simulink model "uplink_8c4r"  (Simulink 8.7)
settings: Solver=VariableStepDiscrete  StartTime=0.0  StopTime=20000  RelTol=1e-3
PreLoadFcn:
  | % Run the setup script when the model is opened
  | setup_uplink_8c4r;
InitFcn:
  | % Run the setup script again just before the
  | % model is run, so that any updates made
  | % after opening are applied.
  | setup_uplink_8c4r;
  | %% DSPBuilder Start
  | alt_dspbuilder_update_model(bdroot)
  | %% DSPBuilder End
undefined symbols (not defined in the file or in its folder): DDC_Lineup_param
libraries: pipereg_lib x8, DSPBABase x7, ddc_mixer_lib x4, hddc_lib x4, lddc_lib x4, simulink x1
Description:
  | DSP Builder Advanced Template for Template Design implementing ModelIP designs
settings Model: Creator=mjervis  LastModifiedBy=5g
settings DataIOCC: SignalLoggingSaveFormat=ModelDataLogs
settings OptimizationCC: ExpressionDepthLimit=2147483647
settings DebuggingCC: SolverPrmCheckMsg=warning  InheritedTsInSrcMsg=none  IntegerOverflowMsg=none  ParameterOverflowMsg=none  FcnCallInpInsideContextMsg=UseLocalSettings  StateNameClashWarn=warning  IntegerSaturationMsg=none
settings GRTTargetCC: CombineOutputUpdateFcns=off  GRTInterface=on
settings ConfigComp: CovSFcnEnable=off

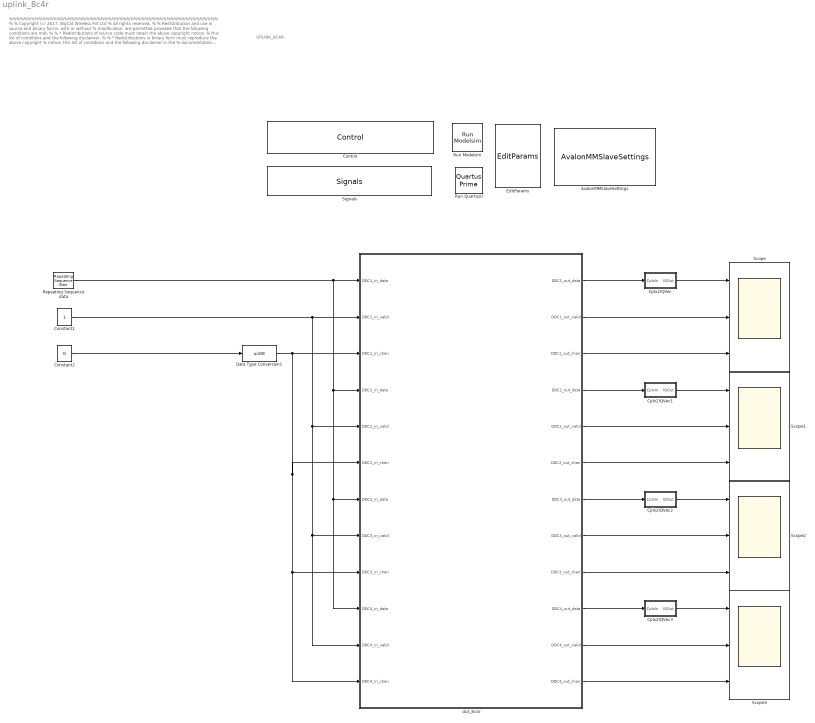
== system uplink_8c4r ==
  note: %%%%%%%%%%%%%%%%%%%%%%%%%%%%%%%%%%%%%%%%%%%%%%%%%%%%%%%%%
      |  %
      |  % Copyright (c) 2017, BigCat Wireless Pvt Ltd
      |  % All rights reserved.
      |  %
      |  % Redistribution and use in source and binary forms, with or without
      |  % modification, are permitted provided that the following conditions are met:
      |  %
      |  %     * Redistributions of source code must retain the above copyright notice,
      |  %       this list of conditions and the following disclaimer.
      |  %
      |  %     * Redistributions in binary form must reproduce the above copyright
      |  %       notice, this list of conditions and the following disclaimer in the
      |  %       documentation and/or other materials provided with the distribution.
      |  %
      |  %     * Neither the name of the copyright holder nor the names of its contributors
      |  %       may be used to endorse or promote products derived from this software
      |  %       without specific prior written permission.
      |  %
      |  %
      |  %
      |  % THIS SOFTWARE IS PROVIDED BY THE COPYRIGHT HOLDERS AND CONTRIBUTORS "AS IS"
      |  % AND ANY EXPRESS OR IMPLIED WARRANTIES, INCLUDING, BUT NOT LIMITED TO, THE
      |  % IMPLIED WARRANTIES OF MERCHANTABILITY AND FITNESS FOR A PARTICULAR PURPOSE ARE
      |  % DISCLAIMED. IN NO EVENT SHALL THE COPYRIGHT HOLDER OR CONTRIBUTORS BE LIABLE
      |  % FOR ANY DIRECT, INDIRECT, INCIDENTAL, SPECIAL, EXEMPLARY, OR CONSEQUENTIAL
      |  % DAMAGES (INCLUDING, BUT NOT LIMITED TO, PROCUREMENT OF SUBSTITUTE GOODS OR
      |  % SERVICES; LOSS OF USE, DATA, OR PROFITS; OR BUSINESS INTERRUPTION) HOWEVER
      |  % CAUSED AND ON ANY THEORY OF LIABILITY, WHETHER IN CONTRACT, STRICT LIABILITY,
      |  % OR TORT (INCLUDING NEGLIGENCE OR OTHERWISE) ARISING IN ANY WAY OUT OF THE USE
      |  % OF THIS SOFTWARE, EVEN IF ADVISED OF THE POSSIBILITY OF SUCH DAMAGE.
      |  %
      |   %%%%%%%%%%%%%%%%%%%%%%%%%%%%%%%%%%%%%%%%%%%%%%%%%%%%%%%%%%
  note: UPLINK_8C4R
  AvalonMMSlaveSettings : DSPBABase/AvalonMMSlaveSettings
  Constant1 : Constant  OutDataTypeStr=boolean
  Constant2 : Constant  Value=0  OutDataTypeStr=boolean
  Control : DSPBABase/Control  generate=on  language=VHDL  destination=./rtl  destination_gui=./rtl  make_full_path=off  path_is_relative=on  autotestbench=off  signaldepth=2  coveragetestbench=on  logs=off  spacewidth=2  spacenum=1  addrwidth=11  datawidth=32  dataendian=Big Endian  hierarchicalnames=off  ramThresholdBits=-1  distRamThresholdBits=-1  mlabThresholdBits=-1  hardMultiplierThresholdLuts=-1  version=20090407  errorOnChanMismatch=1  errorOnGPIOMismatch=0  importModelsimResults=0  cycleAccurate=off  reinterpretCastMult=off  paramFile=uplink_8c4r_params.xml
  Cplx2IQVec : Subsystem
  Cplx2IQVec1 : Subsystem
  Cplx2IQVec2 : Subsystem
  Cplx2IQVec3 : Subsystem
  Data Type Conversion1 : DataTypeConversion  OutDataTypeStr=uint8
  EditParams : DSPBABase/EditParams  version=20090407
  Repeating Sequence data : simulink/Sources/Repeating Sequence Stair  OutValues=DDC_Lineup_param.inputdata.'  tsamp=1  OutMin=[]  OutMax=[]  OutDataTypeStr=fixdt(1,16,15)  OutputDataTypeScalingMode=Specify via dialog  OutDataType=fixdt(1,16,15)  ConRadixGroup=Best Precision: Vector-wise  OutScaling=[]
  Run Modelsim : DSPBABase/Run Modelsim  version=20090407
  "Run QuartusII " : DSPBABase/Quartus Prime  version=20090407
  Scope{,1..3} (4 alike) : Scope  NumInputPorts=3
  Signals : DSPBABase/Signals  clk=clk  freq=DDC_Lineup_param.ClockRate  margin=DDC_Lineup_param.ClockMargin  rst=areset  rstactive=High  bus=bus  enbusclock=on  busfreq=61.44  bussync=on  version=20090407
  dut_8c4r : Subsystem
  wires:
  Constant2/1 -> Data Type Conversion1/1
  Repeating Sequence data/1 -> dut_8c4r/10(DDC4_in_data), dut_8c4r/7(DDC3_in_data), dut_8c4r/4(DDC2_in_data), dut_8c4r/1(DDC1_in_data)
  Constant1/1 -> dut_8c4r/11(DDC4_in_valid), dut_8c4r/8(DDC3_in_valid), dut_8c4r/5(DDC2_in_valid), dut_8c4r/2(DDC1_in_valid)
  Data Type Conversion1/1 -> dut_8c4r/12(DDC4_in_chan), dut_8c4r/9(DDC3_in_chan), dut_8c4r/6(DDC2_in_chan), dut_8c4r/3(DDC1_in_chan)
  dut_8c4r/1(DDC1_out_data) -> Cplx2IQVec/1(CplxIn)
  dut_8c4r/2(DDC1_out_valid) -> Scope/2
  dut_8c4r/3(DDC1_out_chan) -> Scope/3
  dut_8c4r/4(DDC2_out_data) -> Cplx2IQVec1/1(CplxIn)
  dut_8c4r/5(DDC2_out_valid) -> Scope1/2
  dut_8c4r/6(DDC2_out_chan) -> Scope1/3
  dut_8c4r/7(DDC3_out_data) -> Cplx2IQVec2/1(CplxIn)
  dut_8c4r/8(DDC3_out_valid) -> Scope2/2
  dut_8c4r/9(DDC3_out_chan) -> Scope2/3
  dut_8c4r/10(DDC4_out_data) -> Cplx2IQVec3/1(CplxIn)
  dut_8c4r/11(DDC4_out_valid) -> Scope3/2
  dut_8c4r/12(DDC4_out_chan) -> Scope3/3
  Cplx2IQVec/1(IQOut) -> Scope/1
  Cplx2IQVec1/1(IQOut) -> Scope1/1
  Cplx2IQVec2/1(IQOut) -> Scope2/1
  Cplx2IQVec3/1(IQOut) -> Scope3/1

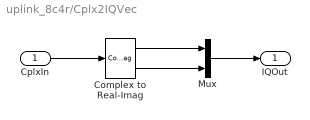
== system uplink_8c4r/Cplx2IQVec ==
  CplxIn : Inport
  Complex to Real-Imag : ComplexToRealImag
  Mux : Mux  Inputs=2
  IQOut : Outport
  wires:
  Complex to Real-Imag/1 -> Mux/1
  Mux/1 -> IQOut/1
  Complex to Real-Imag/2 -> Mux/2
  CplxIn/1 -> Complex to Real-Imag/1

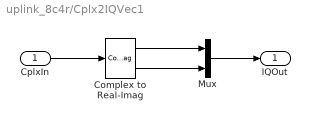
== system uplink_8c4r/Cplx2IQVec1 ==
  CplxIn : Inport
  Complex to Real-Imag : ComplexToRealImag
  Mux : Mux  Inputs=2
  IQOut : Outport
  wires:
  CplxIn/1 -> Complex to Real-Imag/1
  Complex to Real-Imag/2 -> Mux/2
  Mux/1 -> IQOut/1
  Complex to Real-Imag/1 -> Mux/1

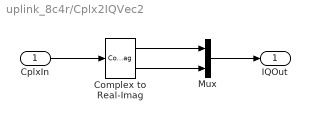
== system uplink_8c4r/Cplx2IQVec2 ==
  CplxIn : Inport
  Complex to Real-Imag : ComplexToRealImag
  Mux : Mux  Inputs=2
  IQOut : Outport
  wires:
  Complex to Real-Imag/1 -> Mux/1
  Mux/1 -> IQOut/1
  Complex to Real-Imag/2 -> Mux/2
  CplxIn/1 -> Complex to Real-Imag/1

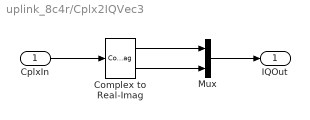
== system uplink_8c4r/Cplx2IQVec3 ==
  CplxIn : Inport
  Complex to Real-Imag : ComplexToRealImag
  Mux : Mux  Inputs=2
  IQOut : Outport
  wires:
  CplxIn/1 -> Complex to Real-Imag/1
  Complex to Real-Imag/2 -> Mux/2
  Mux/1 -> IQOut/1
  Complex to Real-Imag/1 -> Mux/1

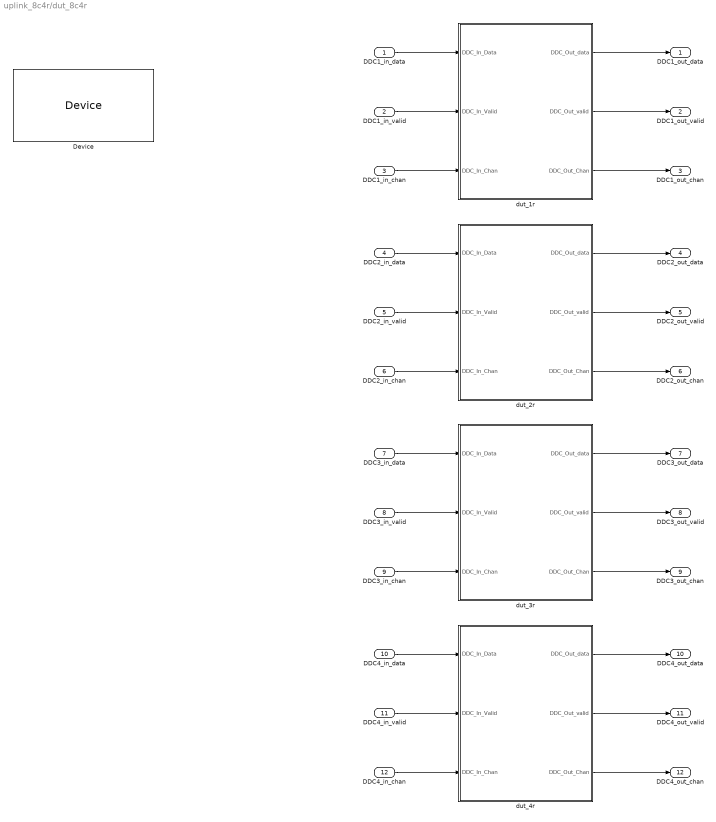
== system uplink_8c4r/dut_8c4r ==
  DDC1_in_data : Inport
  DDC1_in_valid : Inport  Port=2
  DDC1_in_chan : Inport  Port=3
  DDC2_in_data : Inport  Port=4
  DDC2_in_valid : Inport  Port=5
  DDC2_in_chan : Inport  Port=6
  DDC3_in_data : Inport  Port=7
  DDC3_in_valid : Inport  Port=8
  DDC3_in_chan : Inport  Port=9
  DDC4_in_data : Inport  Port=10
  DDC4_in_valid : Inport  Port=11
  DDC4_in_chan : Inport  Port=12
  Device : DSPBABase/Device  family=Arria 10  deviceMember=Arria 10  stratix4device=Stratix IV GX  hardcopy4device=HardCopy IV E  stratix5device=Stratix V GX  device=10AS066N2F40I1SGES  speed=1  stratixSpeed=-5  stratix2Speed=-3  stratix3Speed=-3  stratix4gxSpeed=-2  stratix4gtSpeed=-1  cyclone2Speed=-6  cyclone3Speed=-7  arria2Speed=-4  cyclone4eSpeed=-8  stratix5Speed=-3  arria5Speed=-4  arriaSpeed=-6  cyclone3lsSpeed=-7  cyclone5Speed=-6  arria2gzSpeed=-3  nightFurySpeed=-2  ecp2Speed=-7  hardcopycompat=off  version=20140217  max10flashmode=off  max10nomeminit=off
  dut_1r : Subsystem
  dut_2r : Subsystem
  dut_3r : Subsystem
  dut_4r : Subsystem
  DDC1_out_data : Outport
  DDC1_out_valid : Outport  Port=2
  DDC1_out_chan : Outport  Port=3
  DDC2_out_data : Outport  Port=4
  DDC2_out_valid : Outport  Port=5
  DDC2_out_chan : Outport  Port=6
  DDC3_out_data : Outport  Port=7
  DDC3_out_valid : Outport  Port=8
  DDC3_out_chan : Outport  Port=9
  DDC4_out_data : Outport  Port=10
  DDC4_out_valid : Outport  Port=11
  DDC4_out_chan : Outport  Port=12
  wires:
  dut_1r/1(DDC_Out_data) -> DDC1_out_data/1
  dut_1r/2(DDC_Out_valid) -> DDC1_out_valid/1
  dut_1r/3(DDC_Out_Chan) -> DDC1_out_chan/1
  DDC1_in_data/1 -> dut_1r/1(DDC_In_Data)
  DDC1_in_valid/1 -> dut_1r/2(DDC_In_Valid)
  DDC1_in_chan/1 -> dut_1r/3(DDC_In_Chan)
  dut_2r/1(DDC_Out_data) -> DDC2_out_data/1
  dut_2r/2(DDC_Out_valid) -> DDC2_out_valid/1
  dut_2r/3(DDC_Out_Chan) -> DDC2_out_chan/1
  DDC2_in_data/1 -> dut_2r/1(DDC_In_Data)
  DDC2_in_valid/1 -> dut_2r/2(DDC_In_Valid)
  DDC2_in_chan/1 -> dut_2r/3(DDC_In_Chan)
  dut_3r/1(DDC_Out_data) -> DDC3_out_data/1
  dut_3r/2(DDC_Out_valid) -> DDC3_out_valid/1
  dut_3r/3(DDC_Out_Chan) -> DDC3_out_chan/1
  DDC3_in_data/1 -> dut_3r/1(DDC_In_Data)
  DDC3_in_valid/1 -> dut_3r/2(DDC_In_Valid)
  DDC3_in_chan/1 -> dut_3r/3(DDC_In_Chan)
  dut_4r/1(DDC_Out_data) -> DDC4_out_data/1
  dut_4r/2(DDC_Out_valid) -> DDC4_out_valid/1
  dut_4r/3(DDC_Out_Chan) -> DDC4_out_chan/1
  DDC4_in_data/1 -> dut_4r/1(DDC_In_Data)
  DDC4_in_valid/1 -> dut_4r/2(DDC_In_Valid)
  DDC4_in_chan/1 -> dut_4r/3(DDC_In_Chan)

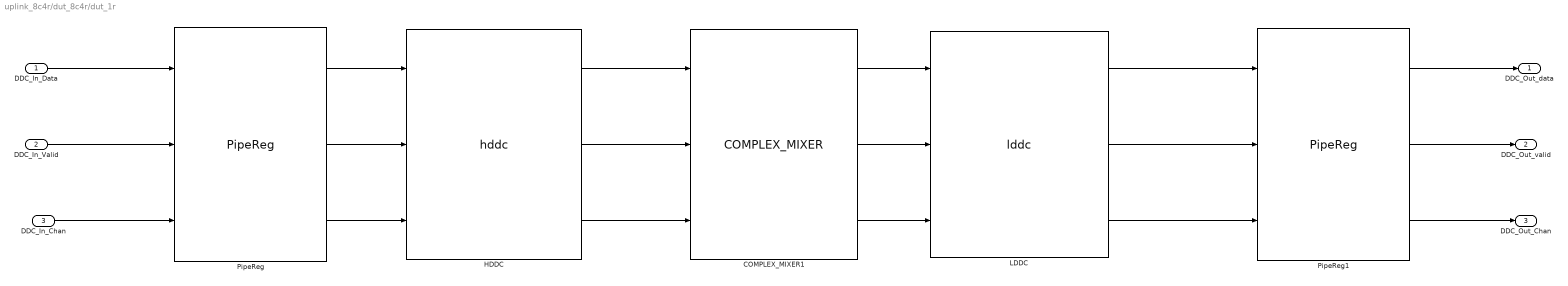
== system uplink_8c4r/dut_8c4r/dut_1r ==
  DDC_In_Data : Inport
  DDC_In_Valid : Inport  Port=2
  DDC_In_Chan : Inport  Port=3
  COMPLEX_MIXER1 : ddc_mixer_lib/COMPLEX_MIXER  CM_pipeline_stages=2  CM_clock_margin=DDC_Lineup_param.ClockMargin  CM_NCO_sample_rate=DDC_Lineup_param.Complex_NCO.SampleRate  CM_NCO_accumulator_bit_width=DDC_Lineup_param.Complex_NCO.Acumulater_bit_wid  CM_NCO_frequency_word=DDC_Lineup_param.Complex_NCO_A1.Freq_word  CM_NCO_base_addr=DDC_Lineup_param.Complex_NCO_A1.base_addr  CM_NCO_data_type=DDC_Lineup_param.Complex_NCO.Data_type  CM_NCO_scaling_value=DDC_Lineup_param.Complex_NCO.scaling_value  CM_sample_rate=DDC_Lineup_param.CM.SampleRate  CM_complex_channels=DDC_Lineup_param.CM.No_Of_complex_chan  CM_complex_freq=DDC_Lineup_param.CM.No_Of_complex_Freq  CM_output_word_length=DDC_Lineup_param.output_word_length  CM_output_fraction_length=DDC_Lineup_param.output_fraction_length  CM_scale_multiplication_factor=DDC_CM_multiplication_factor  CM_scale_left_shift_factor=DDC_CM_Number_of_bits_to_shift_left  CM_NCO_phase=DDC_CM_NCO_phase  CM_NCO_sync=DDC_CM_NCO_sync
      link override ComplexMixer: latency=4
      link override ComplexMixer_Scale: latency=3
      link override ComplexMixer_Scale1: latency=3
      link override Complex_NCO: latency=19
      link override Const2: otype=ufix(2)
      link override NCO Delay Matching/ChannelOut: latency=2
  HDDC : hddc_lib/hddc  Clock_Margin=DDC_Lineup_param.ClockMargin  HB7_filter_SampleRate=DDC_Lineup_param.HB_filter7.SampleRate  HB7_filter_Decimation=DDC_Lineup_param.HB_filter7.Decimation  HB7_filter_ChanCount=DDC_Lineup_param.HB_filter7.ChanCount  HB7_filter_coeffs=DDC_Lineup_param.HB_filt7.coeffs(1,:)  HB7_filter_base_addr=DDC_Lineup_param.HB_filter7.base_addr1  HB6_filter_SampleRate=DDC_Lineup_param.HB_filter6.SampleRate  HB6_filter_Decimation=DDC_Lineup_param.HB_filter6.Decimation  HB6_filter_ChanCount=DDC_Lineup_param.HB_filter6.ChanCount  HB6_filter_coeffs=DDC_Lineup_param.HB_filt6.coeffs(1,:)  HB6_filter_base_addr=DDC_Lineup_param.HB_filter6.base_addr1  output_word_length=DDC_Lineup_param.output_word_length  output_fraction_length=DDC_Lineup_param.output_fraction_length
      link override HB6/HB6Im_Scale: latency=4
      link override HB6/HB6Re_Scale: latency=4
      link override HB6/HB6_Im: latency=13
      link override HB6/HB6_Re: latency=13
      link override HB6/HB_4: latency=14
      link override HB6/HB_4_Scale: latency=6
      link override HB7/HB5_Scale: latency=6
      link override HB7/HB7Im_Scale: latency=4
      link override HB7/HB7Re_Scale: latency=4
      link override HB7/HB7_Im: latency=11
      link override HB7/HB7_Re: latency=11
      link override HB7/HB_5: latency=14
      link override PipeReg1/ChannelOut: value=1  packetBeginEnabled=off  latency=2
      link override PipeReg2/ChannelOut: value=1  packetBeginEnabled=off  latency=2
      link override PipeReg3/ChannelOut: value=1  packetBeginEnabled=off  latency=2
      link override PipeReg4/ChannelOut: value=1  packetBeginEnabled=off  latency=2
  LDDC : lddc_lib/lddc  HB5_filter_SampleRate=DDC_Lineup_param.HB_filter5.SampleRate  HB5_filter_Decimation=DDC_Lineup_param.HB_filter5.Decimation  HB5_filter_ChanCount=DDC_Lineup_param.HB_filter5.ChanCount  HB5_filter_coeffs=DDC_Lineup_param.HB_filt5.coeffs(1,:)  HB5_filter_base_addr=DDC_Lineup_param.HB_filter5.base_addr1  HB4_filter_SampleRate=DDC_Lineup_param.HB_filter4.SampleRate  HB4_filter_Decimation=DDC_Lineup_param.HB_filter4.Decimation  HB4_filter_ChanCount=DDC_Lineup_param.HB_filter4.ChanCount  HB4_filter_coeffs=DDC_Lineup_param.HB_filt4.coeffs(1,:)  HB4_filter_base_addr=DDC_Lineup_param.HB_filter4.base_addr1  CH_filter_SampleRate=DDC_Lineup_param.CH_filter.SampleRate  CH_filter_ChanCount=DDC_Lineup_param.CH_filter.ChanCount  CH_filter_coeffs=DDC_Lineup_param.chan_filter.coeffs(1,:)  CH_filter_base_addr=DDC_Lineup_param.CH_filter.base_addr1  output_word_length=DDC_Lineup_param.output_word_length  output_fraction_length=DDC_Lineup_param.output_fraction_length  Pipeline_stages=2  Clock_Margin=DDC_Lineup_param.ClockMargin
      link override Chan_Filter/chan_filter: latency=4
      link override Chan_Filter/chan_filterIm: latency=22
      link override Chan_Filter/chan_filterIm_Scale: latency=4
      link override Chan_Filter/chan_filterRe: latency=22
      link override Chan_Filter/chan_filterRe_Scale: latency=4
      link override Chan_Filter/chan_filter_Scale: latency=6
      link override HB4/HB4Im: latency=21
      link override HB4/HB4Re: latency=21
      link override HB4/HB_4: latency=29
      link override HB4/HB_4_Scale: latency=6
      link override HB4/scale_HB4Im: latency=4
      link override HB4/scale_HB4Re: latency=4
      link override HB5/HB5Im: latency=20
      link override HB5/HB5Re: latency=20
      link override HB5/HB5_Scale: latency=6
      link override HB5/HB_5: latency=25
      link override HB5/scale_HB5Im: latency=4
      link override HB5/scale_HB5Re: latency=4
      link override PipeReg1/ChannelOut: value=1  packetBeginEnabled=off  latency=2
      link override PipeReg2/ChannelOut: value=1  packetBeginEnabled=off  latency=2
      link override PipeReg3/ChannelOut: value=1  packetBeginEnabled=off  latency=2
      link override PipeReg4/ChannelOut: value=1  packetBeginEnabled=off  latency=2
      link override PipeReg5/ChannelOut: value=1  packetBeginEnabled=off  latency=2
      link override PipeReg6/ChannelOut: value=1  packetBeginEnabled=off  latency=2
  PipeReg : pipereg_lib/PipeReg  NPipe=6  Clock_Margin=DDC_Lineup_param.ClockMargin
      link override ChannelOut: value=1  packetBeginEnabled=off  latency=6
  PipeReg1 : pipereg_lib/PipeReg  NPipe=6  Clock_Margin=DDC_Lineup_param.ClockMargin
      link override ChannelOut: value=1  packetBeginEnabled=off  latency=6
  DDC_Out_data : Outport
  DDC_Out_valid : Outport  Port=2
  DDC_Out_Chan : Outport  Port=3
  wires:
  DDC_In_Valid/1 -> PipeReg/2
  DDC_In_Chan/1 -> PipeReg/3
  DDC_In_Data/1 -> PipeReg/1
  PipeReg1/1 -> DDC_Out_data/1
  PipeReg1/2 -> DDC_Out_valid/1
  PipeReg1/3 -> DDC_Out_Chan/1
  LDDC/1 -> PipeReg1/1
  LDDC/2 -> PipeReg1/2
  LDDC/3 -> PipeReg1/3
  PipeReg/2 -> HDDC/2
  PipeReg/3 -> HDDC/3
  PipeReg/1 -> HDDC/1
  COMPLEX_MIXER1/1 -> LDDC/1
  COMPLEX_MIXER1/2 -> LDDC/2
  COMPLEX_MIXER1/3 -> LDDC/3
  HDDC/1 -> COMPLEX_MIXER1/1
  HDDC/2 -> COMPLEX_MIXER1/2
  HDDC/3 -> COMPLEX_MIXER1/3

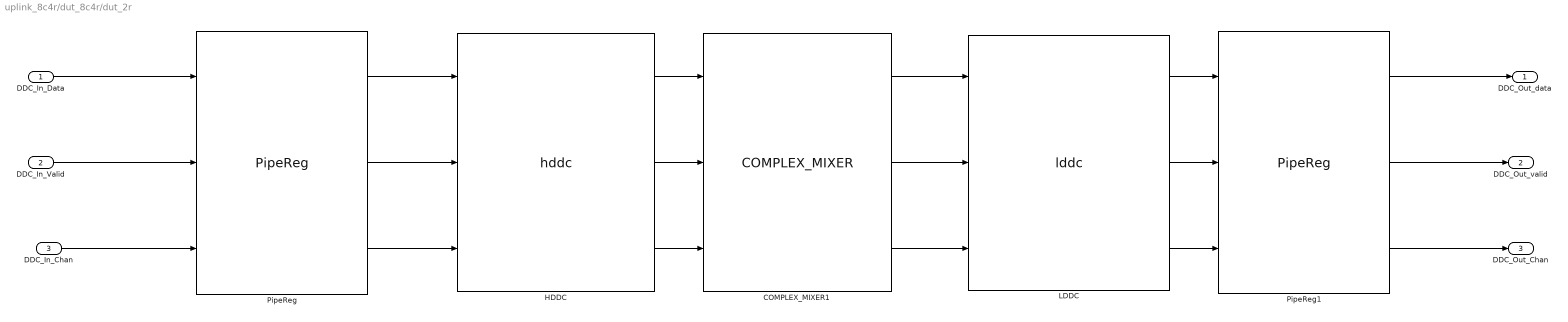
== system uplink_8c4r/dut_8c4r/dut_2r ==
  DDC_In_Data : Inport
  DDC_In_Valid : Inport  Port=2
  DDC_In_Chan : Inport  Port=3
  COMPLEX_MIXER1 : ddc_mixer_lib/COMPLEX_MIXER  CM_pipeline_stages=2  CM_clock_margin=DDC_Lineup_param.ClockMargin  CM_NCO_sample_rate=DDC_Lineup_param.Complex_NCO.SampleRate  CM_NCO_accumulator_bit_width=DDC_Lineup_param.Complex_NCO.Acumulater_bit_wid  CM_NCO_frequency_word=DDC_Lineup_param.Complex_NCO_A2.Freq_word  CM_NCO_base_addr=DDC_Lineup_param.Complex_NCO_A2.base_addr  CM_NCO_data_type=DDC_Lineup_param.Complex_NCO.Data_type  CM_NCO_scaling_value=DDC_Lineup_param.Complex_NCO.scaling_value  CM_sample_rate=DDC_Lineup_param.CM.SampleRate  CM_complex_channels=DDC_Lineup_param.CM.No_Of_complex_chan  CM_complex_freq=DDC_Lineup_param.CM.No_Of_complex_Freq  CM_output_word_length=DDC_Lineup_param.output_word_length  CM_output_fraction_length=DDC_Lineup_param.output_fraction_length  CM_scale_multiplication_factor=DDC_CM_multiplication_factor  CM_scale_left_shift_factor=DDC_CM_Number_of_bits_to_shift_left  CM_NCO_phase=DDC_CM_NCO_phase  CM_NCO_sync=DDC_CM_NCO_sync
      link override ComplexMixer: latency=4
      link override ComplexMixer_Scale: latency=3
      link override ComplexMixer_Scale1: latency=3
      link override Complex_NCO: latency=19
      link override Const2: otype=ufix(2)
      link override NCO Delay Matching/ChannelOut: latency=2
  HDDC : hddc_lib/hddc  Clock_Margin=DDC_Lineup_param.ClockMargin  HB7_filter_SampleRate=DDC_Lineup_param.HB_filter7.SampleRate  HB7_filter_Decimation=DDC_Lineup_param.HB_filter7.Decimation  HB7_filter_ChanCount=DDC_Lineup_param.HB_filter7.ChanCount  HB7_filter_coeffs=DDC_Lineup_param.HB_filt7.coeffs(1,:)  HB7_filter_base_addr=DDC_Lineup_param.HB_filter7.base_addr2  HB6_filter_SampleRate=DDC_Lineup_param.HB_filter6.SampleRate  HB6_filter_Decimation=DDC_Lineup_param.HB_filter6.Decimation  HB6_filter_ChanCount=DDC_Lineup_param.HB_filter6.ChanCount  HB6_filter_coeffs=DDC_Lineup_param.HB_filt6.coeffs(1,:)  HB6_filter_base_addr=DDC_Lineup_param.HB_filter6.base_addr2  output_word_length=DDC_Lineup_param.output_word_length  output_fraction_length=DDC_Lineup_param.output_fraction_length
      link override HB6/HB6Im_Scale: latency=4
      link override HB6/HB6Re_Scale: latency=4
      link override HB6/HB6_Im: latency=13
      link override HB6/HB6_Re: latency=13
      link override HB6/HB_4: latency=14
      link override HB6/HB_4_Scale: latency=6
      link override HB7/HB5_Scale: latency=6
      link override HB7/HB7Im_Scale: latency=4
      link override HB7/HB7Re_Scale: latency=4
      link override HB7/HB7_Im: latency=11
      link override HB7/HB7_Re: latency=11
      link override HB7/HB_5: latency=14
      link override PipeReg1/ChannelOut: value=1  packetBeginEnabled=off  latency=2
      link override PipeReg2/ChannelOut: value=1  packetBeginEnabled=off  latency=2
      link override PipeReg3/ChannelOut: value=1  packetBeginEnabled=off  latency=2
      link override PipeReg4/ChannelOut: value=1  packetBeginEnabled=off  latency=2
  LDDC : lddc_lib/lddc  HB5_filter_SampleRate=DDC_Lineup_param.HB_filter5.SampleRate  HB5_filter_Decimation=DDC_Lineup_param.HB_filter5.Decimation  HB5_filter_ChanCount=DDC_Lineup_param.HB_filter5.ChanCount  HB5_filter_coeffs=DDC_Lineup_param.HB_filt5.coeffs(1,:)  HB5_filter_base_addr=DDC_Lineup_param.HB_filter5.base_addr2  HB4_filter_SampleRate=DDC_Lineup_param.HB_filter4.SampleRate  HB4_filter_Decimation=DDC_Lineup_param.HB_filter4.Decimation  HB4_filter_ChanCount=DDC_Lineup_param.HB_filter4.ChanCount  HB4_filter_coeffs=DDC_Lineup_param.HB_filt4.coeffs(1,:)  HB4_filter_base_addr=DDC_Lineup_param.HB_filter4.base_addr2  CH_filter_SampleRate=DDC_Lineup_param.CH_filter.SampleRate  CH_filter_ChanCount=DDC_Lineup_param.CH_filter.ChanCount  CH_filter_coeffs=DDC_Lineup_param.chan_filter.coeffs(1,:)  CH_filter_base_addr=DDC_Lineup_param.CH_filter.base_addr2  output_word_length=DDC_Lineup_param.output_word_length  output_fraction_length=DDC_Lineup_param.output_fraction_length  Pipeline_stages=2  Clock_Margin=DDC_Lineup_param.ClockMargin
      link override Chan_Filter/chan_filter: latency=4
      link override Chan_Filter/chan_filterIm: latency=22
      link override Chan_Filter/chan_filterIm_Scale: latency=4
      link override Chan_Filter/chan_filterRe: latency=22
      link override Chan_Filter/chan_filterRe_Scale: latency=4
      link override Chan_Filter/chan_filter_Scale: latency=6
      link override HB4/HB4Im: latency=21
      link override HB4/HB4Re: latency=21
      link override HB4/HB_4: latency=29
      link override HB4/HB_4_Scale: latency=6
      link override HB4/scale_HB4Im: latency=4
      link override HB4/scale_HB4Re: latency=4
      link override HB5/HB5Im: latency=20
      link override HB5/HB5Re: latency=20
      link override HB5/HB5_Scale: latency=6
      link override HB5/HB_5: latency=25
      link override HB5/scale_HB5Im: latency=4
      link override HB5/scale_HB5Re: latency=4
      link override PipeReg1/ChannelOut: value=1  packetBeginEnabled=off  latency=2
      link override PipeReg2/ChannelOut: value=1  packetBeginEnabled=off  latency=2
      link override PipeReg3/ChannelOut: value=1  packetBeginEnabled=off  latency=2
      link override PipeReg4/ChannelOut: value=1  packetBeginEnabled=off  latency=2
      link override PipeReg5/ChannelOut: value=1  packetBeginEnabled=off  latency=2
      link override PipeReg6/ChannelOut: value=1  packetBeginEnabled=off  latency=2
  PipeReg : pipereg_lib/PipeReg  NPipe=6  Clock_Margin=DDC_Lineup_param.ClockMargin
      link override ChannelOut: value=1  packetBeginEnabled=off  latency=6
  PipeReg1 : pipereg_lib/PipeReg  NPipe=6  Clock_Margin=DDC_Lineup_param.ClockMargin
      link override ChannelOut: value=1  packetBeginEnabled=off  latency=6
  DDC_Out_data : Outport
  DDC_Out_valid : Outport  Port=2
  DDC_Out_Chan : Outport  Port=3
  wires:
  DDC_In_Valid/1 -> PipeReg/2
  DDC_In_Chan/1 -> PipeReg/3
  DDC_In_Data/1 -> PipeReg/1
  PipeReg1/1 -> DDC_Out_data/1
  PipeReg1/2 -> DDC_Out_valid/1
  PipeReg1/3 -> DDC_Out_Chan/1
  HDDC/1 -> COMPLEX_MIXER1/1
  HDDC/2 -> COMPLEX_MIXER1/2
  HDDC/3 -> COMPLEX_MIXER1/3
  COMPLEX_MIXER1/1 -> LDDC/1
  COMPLEX_MIXER1/2 -> LDDC/2
  COMPLEX_MIXER1/3 -> LDDC/3
  LDDC/1 -> PipeReg1/1
  LDDC/2 -> PipeReg1/2
  LDDC/3 -> PipeReg1/3
  PipeReg/2 -> HDDC/2
  PipeReg/3 -> HDDC/3
  PipeReg/1 -> HDDC/1

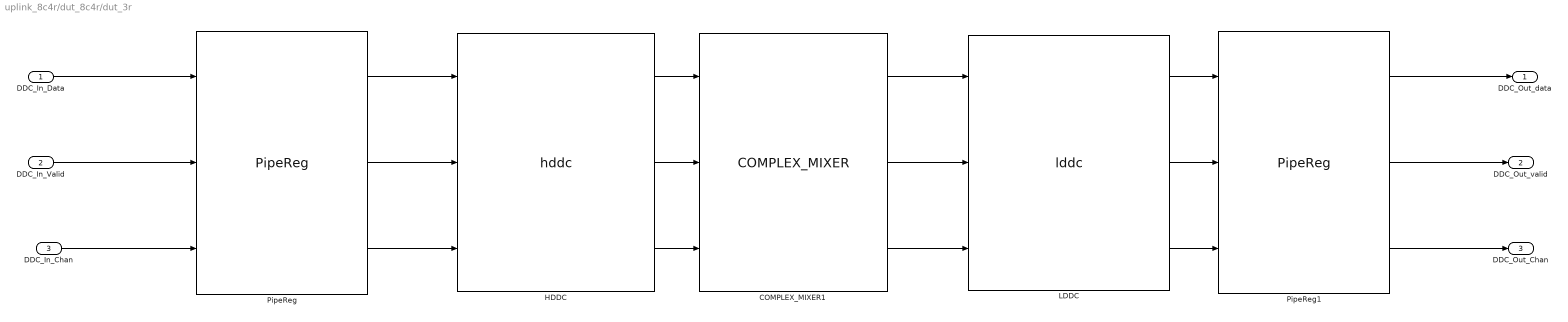
== system uplink_8c4r/dut_8c4r/dut_3r ==
  DDC_In_Data : Inport
  DDC_In_Valid : Inport  Port=2
  DDC_In_Chan : Inport  Port=3
  COMPLEX_MIXER1 : ddc_mixer_lib/COMPLEX_MIXER  CM_pipeline_stages=2  CM_clock_margin=DDC_Lineup_param.ClockMargin  CM_NCO_sample_rate=DDC_Lineup_param.Complex_NCO.SampleRate  CM_NCO_accumulator_bit_width=DDC_Lineup_param.Complex_NCO.Acumulater_bit_wid  CM_NCO_frequency_word=DDC_Lineup_param.Complex_NCO_A3.Freq_word  CM_NCO_base_addr=DDC_Lineup_param.Complex_NCO_A3.base_addr  CM_NCO_data_type=DDC_Lineup_param.Complex_NCO.Data_type  CM_NCO_scaling_value=DDC_Lineup_param.Complex_NCO.scaling_value  CM_sample_rate=DDC_Lineup_param.CM.SampleRate  CM_complex_channels=DDC_Lineup_param.CM.No_Of_complex_chan  CM_complex_freq=DDC_Lineup_param.CM.No_Of_complex_Freq  CM_output_word_length=DDC_Lineup_param.output_word_length  CM_output_fraction_length=DDC_Lineup_param.output_fraction_length  CM_scale_multiplication_factor=DDC_CM_multiplication_factor  CM_scale_left_shift_factor=DDC_CM_Number_of_bits_to_shift_left  CM_NCO_phase=DDC_CM_NCO_phase  CM_NCO_sync=DDC_CM_NCO_sync
      link override ComplexMixer: latency=4
      link override ComplexMixer_Scale: latency=3
      link override ComplexMixer_Scale1: latency=3
      link override Complex_NCO: latency=19
      link override Const2: scale=1  otype=ufix(2)
      link override NCO Delay Matching/ChannelOut: latency=2
  HDDC : hddc_lib/hddc  Clock_Margin=DDC_Lineup_param.ClockMargin  HB7_filter_SampleRate=DDC_Lineup_param.HB_filter7.SampleRate  HB7_filter_Decimation=DDC_Lineup_param.HB_filter7.Decimation  HB7_filter_ChanCount=DDC_Lineup_param.HB_filter7.ChanCount  HB7_filter_coeffs=DDC_Lineup_param.HB_filt7.coeffs(1,:)  HB7_filter_base_addr=DDC_Lineup_param.HB_filter7.base_addr3  HB6_filter_SampleRate=DDC_Lineup_param.HB_filter6.SampleRate  HB6_filter_Decimation=DDC_Lineup_param.HB_filter6.Decimation  HB6_filter_ChanCount=DDC_Lineup_param.HB_filter6.ChanCount  HB6_filter_coeffs=DDC_Lineup_param.HB_filt6.coeffs(1,:)  HB6_filter_base_addr=DDC_Lineup_param.HB_filter6.base_addr3  output_word_length=DDC_Lineup_param.output_word_length  output_fraction_length=DDC_Lineup_param.output_fraction_length
      link override HB6/HB6Im_Scale: latency=4
      link override HB6/HB6Re_Scale: latency=4
      link override HB6/HB6_Im: latency=13
      link override HB6/HB6_Re: latency=13
      link override HB6/HB_4: latency=14
      link override HB6/HB_4_Scale: latency=6
      link override HB7/HB5_Scale: latency=6
      link override HB7/HB7Im_Scale: latency=4
      link override HB7/HB7Re_Scale: latency=4
      link override HB7/HB7_Im: latency=11
      link override HB7/HB7_Re: latency=11
      link override HB7/HB_5: latency=14
      link override PipeReg1/ChannelOut: value=1  packetBeginEnabled=off  latency=2
      link override PipeReg2/ChannelOut: value=1  packetBeginEnabled=off  latency=2
      link override PipeReg3/ChannelOut: value=1  packetBeginEnabled=off  latency=2
      link override PipeReg4/ChannelOut: value=1  packetBeginEnabled=off  latency=2
  LDDC : lddc_lib/lddc  HB5_filter_SampleRate=DDC_Lineup_param.HB_filter5.SampleRate  HB5_filter_Decimation=DDC_Lineup_param.HB_filter5.Decimation  HB5_filter_ChanCount=DDC_Lineup_param.HB_filter5.ChanCount  HB5_filter_coeffs=DDC_Lineup_param.HB_filt5.coeffs(1,:)  HB5_filter_base_addr=DDC_Lineup_param.HB_filter5.base_addr3  HB4_filter_SampleRate=DDC_Lineup_param.HB_filter4.SampleRate  HB4_filter_Decimation=DDC_Lineup_param.HB_filter4.Decimation  HB4_filter_ChanCount=DDC_Lineup_param.HB_filter4.ChanCount  HB4_filter_coeffs=DDC_Lineup_param.HB_filt4.coeffs(1,:)  HB4_filter_base_addr=DDC_Lineup_param.HB_filter4.base_addr3  CH_filter_SampleRate=DDC_Lineup_param.CH_filter.SampleRate  CH_filter_ChanCount=DDC_Lineup_param.CH_filter.ChanCount  CH_filter_coeffs=DDC_Lineup_param.chan_filter.coeffs(1,:)  CH_filter_base_addr=DDC_Lineup_param.CH_filter.base_addr3  output_word_length=DDC_Lineup_param.output_word_length  output_fraction_length=DDC_Lineup_param.output_fraction_length  Pipeline_stages=2  Clock_Margin=DDC_Lineup_param.ClockMargin
      link override Chan_Filter/chan_filter: latency=4
      link override Chan_Filter/chan_filterIm: latency=22
      link override Chan_Filter/chan_filterIm_Scale: latency=4
      link override Chan_Filter/chan_filterRe: latency=22
      link override Chan_Filter/chan_filterRe_Scale: latency=4
      link override Chan_Filter/chan_filter_Scale: latency=6
      link override HB4/HB4Im: latency=21
      link override HB4/HB4Re: latency=21
      link override HB4/HB_4: latency=29
      link override HB4/HB_4_Scale: latency=6
      link override HB4/scale_HB4Im: latency=4
      link override HB4/scale_HB4Re: latency=4
      link override HB5/HB5Im: latency=20
      link override HB5/HB5Re: latency=20
      link override HB5/HB5_Scale: latency=6
      link override HB5/HB_5: latency=25
      link override HB5/scale_HB5Im: latency=4
      link override HB5/scale_HB5Re: latency=4
      link override PipeReg1/ChannelOut: value=1  packetBeginEnabled=off  latency=2
      link override PipeReg2/ChannelOut: value=1  packetBeginEnabled=off  latency=2
      link override PipeReg3/ChannelOut: value=1  packetBeginEnabled=off  latency=2
      link override PipeReg4/ChannelOut: value=1  packetBeginEnabled=off  latency=2
      link override PipeReg5/ChannelOut: value=1  packetBeginEnabled=off  latency=2
      link override PipeReg6/ChannelOut: value=1  packetBeginEnabled=off  latency=2
  PipeReg : pipereg_lib/PipeReg  NPipe=6  Clock_Margin=DDC_Lineup_param.ClockMargin
      link override ChannelOut: value=1  packetBeginEnabled=off  latency=6
  PipeReg1 : pipereg_lib/PipeReg  NPipe=6  Clock_Margin=DDC_Lineup_param.ClockMargin
      link override ChannelOut: value=1  packetBeginEnabled=off  latency=6
  DDC_Out_data : Outport
  DDC_Out_valid : Outport  Port=2
  DDC_Out_Chan : Outport  Port=3
  wires:
  DDC_In_Valid/1 -> PipeReg/2
  DDC_In_Chan/1 -> PipeReg/3
  DDC_In_Data/1 -> PipeReg/1
  PipeReg1/1 -> DDC_Out_data/1
  PipeReg1/2 -> DDC_Out_valid/1
  PipeReg1/3 -> DDC_Out_Chan/1
  HDDC/1 -> COMPLEX_MIXER1/1
  HDDC/2 -> COMPLEX_MIXER1/2
  HDDC/3 -> COMPLEX_MIXER1/3
  COMPLEX_MIXER1/1 -> LDDC/1
  COMPLEX_MIXER1/2 -> LDDC/2
  COMPLEX_MIXER1/3 -> LDDC/3
  LDDC/1 -> PipeReg1/1
  LDDC/2 -> PipeReg1/2
  LDDC/3 -> PipeReg1/3
  PipeReg/2 -> HDDC/2
  PipeReg/3 -> HDDC/3
  PipeReg/1 -> HDDC/1

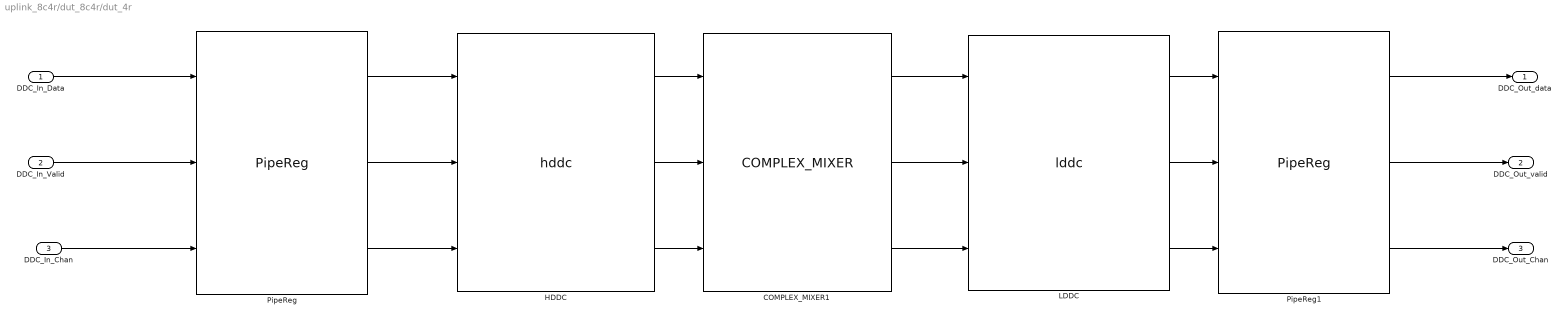
== system uplink_8c4r/dut_8c4r/dut_4r ==
  DDC_In_Data : Inport
  DDC_In_Valid : Inport  Port=2
  DDC_In_Chan : Inport  Port=3
  COMPLEX_MIXER1 : ddc_mixer_lib/COMPLEX_MIXER  CM_pipeline_stages=2  CM_clock_margin=DDC_Lineup_param.ClockMargin  CM_NCO_sample_rate=DDC_Lineup_param.Complex_NCO.SampleRate  CM_NCO_accumulator_bit_width=DDC_Lineup_param.Complex_NCO.Acumulater_bit_wid  CM_NCO_frequency_word=DDC_Lineup_param.Complex_NCO_A4.Freq_word  CM_NCO_base_addr=DDC_Lineup_param.Complex_NCO_A4.base_addr  CM_NCO_data_type=DDC_Lineup_param.Complex_NCO.Data_type  CM_NCO_scaling_value=DDC_Lineup_param.Complex_NCO.scaling_value  CM_sample_rate=DDC_Lineup_param.CM.SampleRate  CM_complex_channels=DDC_Lineup_param.CM.No_Of_complex_chan  CM_complex_freq=DDC_Lineup_param.CM.No_Of_complex_Freq  CM_output_word_length=DDC_Lineup_param.output_word_length  CM_output_fraction_length=DDC_Lineup_param.output_fraction_length  CM_scale_multiplication_factor=DDC_CM_multiplication_factor  CM_scale_left_shift_factor=DDC_CM_Number_of_bits_to_shift_left  CM_NCO_phase=DDC_CM_NCO_phase  CM_NCO_sync=DDC_CM_NCO_sync
      link override ComplexMixer: latency=4
      link override ComplexMixer_Scale: latency=3
      link override ComplexMixer_Scale1: latency=3
      link override Complex_NCO: latency=19
      link override Const2: otype=ufix(2)
      link override NCO Delay Matching/ChannelOut: latency=2
  HDDC : hddc_lib/hddc  Clock_Margin=DDC_Lineup_param.ClockMargin  HB7_filter_SampleRate=DDC_Lineup_param.HB_filter7.SampleRate  HB7_filter_Decimation=DDC_Lineup_param.HB_filter7.Decimation  HB7_filter_ChanCount=DDC_Lineup_param.HB_filter7.ChanCount  HB7_filter_coeffs=DDC_Lineup_param.HB_filt7.coeffs(1,:)  HB7_filter_base_addr=DDC_Lineup_param.HB_filter7.base_addr4  HB6_filter_SampleRate=DDC_Lineup_param.HB_filter6.SampleRate  HB6_filter_Decimation=DDC_Lineup_param.HB_filter6.Decimation  HB6_filter_ChanCount=DDC_Lineup_param.HB_filter6.ChanCount  HB6_filter_coeffs=DDC_Lineup_param.HB_filt6.coeffs(1,:)  HB6_filter_base_addr=DDC_Lineup_param.HB_filter6.base_addr4  output_word_length=DDC_Lineup_param.output_word_length  output_fraction_length=DDC_Lineup_param.output_fraction_length
      link override HB6/HB6Im_Scale: latency=4
      link override HB6/HB6Re_Scale: latency=4
      link override HB6/HB6_Im: latency=13
      link override HB6/HB6_Re: latency=13
      link override HB6/HB_4: latency=14
      link override HB6/HB_4_Scale: latency=6
      link override HB7/HB5_Scale: latency=6
      link override HB7/HB7Im_Scale: latency=4
      link override HB7/HB7Re_Scale: latency=4
      link override HB7/HB7_Im: latency=11
      link override HB7/HB7_Re: latency=11
      link override HB7/HB_5: latency=14
      link override PipeReg1/ChannelOut: value=1  packetBeginEnabled=off  latency=2
      link override PipeReg2/ChannelOut: value=1  packetBeginEnabled=off  latency=2
      link override PipeReg3/ChannelOut: value=1  packetBeginEnabled=off  latency=2
      link override PipeReg4/ChannelOut: value=1  packetBeginEnabled=off  latency=2
  LDDC : lddc_lib/lddc  HB5_filter_SampleRate=DDC_Lineup_param.HB_filter5.SampleRate  HB5_filter_Decimation=DDC_Lineup_param.HB_filter5.Decimation  HB5_filter_ChanCount=DDC_Lineup_param.HB_filter5.ChanCount  HB5_filter_coeffs=DDC_Lineup_param.HB_filt5.coeffs(1,:)  HB5_filter_base_addr=DDC_Lineup_param.HB_filter5.base_addr4  HB4_filter_SampleRate=DDC_Lineup_param.HB_filter4.SampleRate  HB4_filter_Decimation=DDC_Lineup_param.HB_filter4.Decimation  HB4_filter_ChanCount=DDC_Lineup_param.HB_filter4.ChanCount  HB4_filter_coeffs=DDC_Lineup_param.HB_filt4.coeffs(1,:)  HB4_filter_base_addr=DDC_Lineup_param.HB_filter4.base_addr4  CH_filter_SampleRate=DDC_Lineup_param.CH_filter.SampleRate  CH_filter_ChanCount=DDC_Lineup_param.CH_filter.ChanCount  CH_filter_coeffs=DDC_Lineup_param.chan_filter.coeffs(1,:)  CH_filter_base_addr=DDC_Lineup_param.CH_filter.base_addr4  output_word_length=DDC_Lineup_param.output_word_length  output_fraction_length=DDC_Lineup_param.output_fraction_length  Pipeline_stages=2  Clock_Margin=DDC_Lineup_param.ClockMargin
      link override Chan_Filter/chan_filter: latency=4
      link override Chan_Filter/chan_filterIm: latency=22
      link override Chan_Filter/chan_filterIm_Scale: latency=4
      link override Chan_Filter/chan_filterRe: latency=22
      link override Chan_Filter/chan_filterRe_Scale: latency=4
      link override Chan_Filter/chan_filter_Scale: latency=6
      link override HB4/HB4Im: latency=21
      link override HB4/HB4Re: latency=21
      link override HB4/HB_4: latency=29
      link override HB4/HB_4_Scale: latency=6
      link override HB4/scale_HB4Im: latency=4
      link override HB4/scale_HB4Re: latency=4
      link override HB5/HB5Im: latency=20
      link override HB5/HB5Re: latency=20
      link override HB5/HB5_Scale: latency=6
      link override HB5/HB_5: latency=25
      link override HB5/scale_HB5Im: latency=4
      link override HB5/scale_HB5Re: latency=4
      link override PipeReg1/ChannelOut: value=1  packetBeginEnabled=off  latency=2
      link override PipeReg2/ChannelOut: value=1  packetBeginEnabled=off  latency=2
      link override PipeReg3/ChannelOut: value=1  packetBeginEnabled=off  latency=2
      link override PipeReg4/ChannelOut: value=1  packetBeginEnabled=off  latency=2
      link override PipeReg5/ChannelOut: value=1  packetBeginEnabled=off  latency=2
      link override PipeReg6/ChannelOut: value=1  packetBeginEnabled=off  latency=2
  PipeReg : pipereg_lib/PipeReg  NPipe=6  Clock_Margin=DDC_Lineup_param.ClockMargin
      link override ChannelOut: value=1  packetBeginEnabled=off  latency=6
  PipeReg1 : pipereg_lib/PipeReg  NPipe=6  Clock_Margin=DDC_Lineup_param.ClockMargin
      link override ChannelOut: value=1  packetBeginEnabled=off  latency=6
  DDC_Out_data : Outport
  DDC_Out_valid : Outport  Port=2
  DDC_Out_Chan : Outport  Port=3
  wires:
  DDC_In_Valid/1 -> PipeReg/2
  DDC_In_Chan/1 -> PipeReg/3
  DDC_In_Data/1 -> PipeReg/1
  PipeReg1/1 -> DDC_Out_data/1
  PipeReg1/2 -> DDC_Out_valid/1
  PipeReg1/3 -> DDC_Out_Chan/1
  HDDC/1 -> COMPLEX_MIXER1/1
  HDDC/2 -> COMPLEX_MIXER1/2
  HDDC/3 -> COMPLEX_MIXER1/3
  COMPLEX_MIXER1/1 -> LDDC/1
  COMPLEX_MIXER1/2 -> LDDC/2
  COMPLEX_MIXER1/3 -> LDDC/3
  LDDC/1 -> PipeReg1/1
  LDDC/2 -> PipeReg1/2
  LDDC/3 -> PipeReg1/3
  PipeReg/2 -> HDDC/2
  PipeReg/3 -> HDDC/3
  PipeReg/1 -> HDDC/1
